simulink model "driver"  (R2013a)
settings: Solver=ode3  SolverMode=SingleTasking  StartTime=0.0  StopTime=inf  RelTol=1e-3
StartFcn:
  | %The GUI handles are by default hidden, turn them on
  | set(0,'ShowHiddenHandles','on');
  | 
  | %event listener for color detector
  | blk = 'driver/Color Detector/detector';
  | event = 'PostOutputs';
  | listener = @update_gui_circle_detect;
  | h = add_exec_event_listener(blk, event, listener);
  | 
  | %event listener for steering angle (manual drive)
  | blk2 = 'driver/Encoder1';
  | event2 = 'PostOutputs';
  | listener2 = @update_gui_steer_angle;
  | h2 = add_exec_event_listener(blk2, event2, listener2);
  | 
  | %event listener for pose updates
  | blk3 = 'driver/Dead Reckoning/Bicycle Model/Pose Integrator';
  | event3 = 'PostOutputs';
  | listener3 = @update_gui_robot_pose;
  | h3 = add_exec_event_listener(blk3, event3, listener3);
undefined symbols (not defined in the file or in its folder): Normalized, PARAMS
libraries: legonxtlib x8, simulink x1
settings Model: SimulationMode=external  ExtModeTrigDuration=2  Creator=anton  LastModifiedBy=anton
settings OptimizationCC: OptimizeModelRefInitCode=on  LifeSpan=1
settings DebuggingCC: SolverPrmCheckMsg=none  StrictBusMsg=Warning
settings HardwareCC: ProdLargestAtomicInteger=Long  ProdLargestAtomicFloat=Float  ProdEndianess=LittleEndian  ProdHWDeviceType=ARM Compatible->ARM 7
settings RTWCC: SystemTargetFile=realtime.tlc  GenerateMakefile=off  TemplateMakefile=realtime.tmf  Description=Run on Target Hardware  RTWVerbose=off  ProcessScript=realtime_make_rtw_hook
settings STFCustomTargetCC: TargetLibSuffix=.a  GenerateSampleERTMain=on  ERTCustomFileBanners=on  SupportNonInlinedSFcns=off  SupportVariableSizeSignals=on  MATLABClassNameForMDSCustomization=Simulink.SoftwareTarget.ERTCustomization  SystemTargetFile=realtime.tlc
settings ERTTargetCC: ParMdlRefBuildCompliant=off  CompOptLevelCompliant=off  ConcurrentExecutionCompliant=off  CombineOutputUpdateFcns=off  ERTFirstTimeCompliant=off  SupportContinuousTime=on  SupportVariableSizeSignals=on  ModelStepFunctionPrototypeControlCompliant=off  CPPClassGenCompliant=off  ExtMode=on  ExtModeTransport=2  ExtModeMexFile=ext_serial_win32_comm_no_acks_rtt  ExtModeMexArgs=0 5 9600  ERTSrcFileBannerTemplate=realtime_code_template.cgt  ERTHdrFileBannerTemplate=realtime_code_template.cgt  ERTDataSrcFileTemplate=realtime_code_template.cgt  ERTDataHdrFileTemplate=realtime_code_template.cgt  ERTCustomFileTemplate=realtime_file_process.tlc

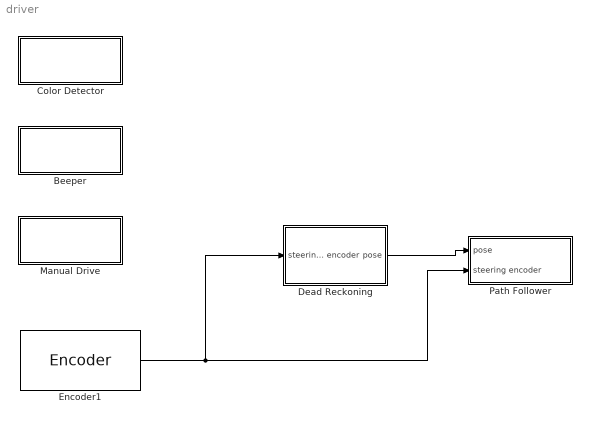
== system driver ==
  Beeper : Subsystem
  Color Detector : Subsystem
  Dead Reckoning : Subsystem
  Encoder1 : legonxtlib/Encoder  portNumber=A  opMode=No reset  sampleTime=0.01
  Manual Drive : Subsystem
  Path Follower : Subsystem
  wires:
  Dead Reckoning/1(pose) -> Path Follower/1(pose)
  Encoder1/1 -> Path Follower/2(steering encoder), Dead Reckoning/1(steering encoder)

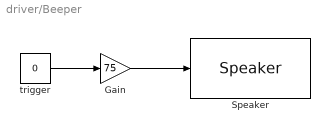
== system driver/Beeper ==
  Gain : Gain  Gain=75
  Speaker : legonxtlib/Speaker  sinputMode=Volume only  sspeakerFreq=440  sspeakerVolume=50  sspeakerDuration=50
  trigger : Constant  Value=0
  wires:
  Gain/1 -> Speaker/1
  trigger/1 -> Gain/1

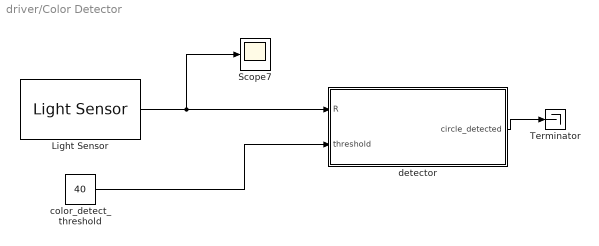
== system driver/Color Detector ==
  Light Sensor : legonxtlib/Light Sensor  portNumber=1  outputMode=Normalized (0 -100)  lightOn=on  sampleTime=0.1
  Scope7 : Scope
      settings: YMin=25  YMax=65
  Terminator : Terminator
  color_detect_threshold : Constant  Value=40
  detector : MATLAB Function  TreatAsAtomicUnit=on
  wires:
  detector/1(circle_detected) -> Terminator/1
  color_detect_threshold/1 -> detector/2(threshold)
  Light Sensor/1 -> Scope7/1, detector/1(R)

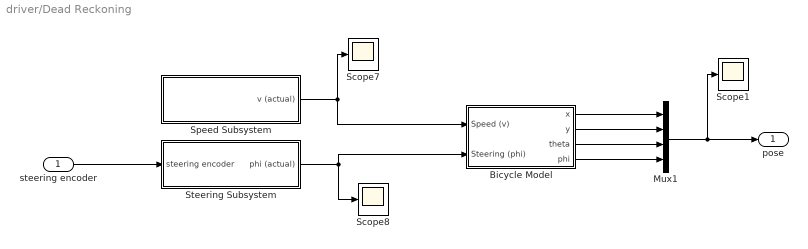
== system driver/Dead Reckoning ==
  steering encoder : Inport
  Bicycle Model : Subsystem
  Mux1 : Mux
  Scope1 : Scope
      settings: YMin=0  YMax=0.95
  Scope7 : Scope
      settings: YMin=0  YMax=14  SaveName=ScopeData19
  Scope8 : Scope
      settings: YMin=0.0523599  YMax=0.0523599  SaveName=ScopeData20
  Speed Subsystem : Subsystem
  Steering Subsystem : Subsystem
  pose : Outport
  wires:
  Bicycle Model/2(y) -> Mux1/2
  Bicycle Model/1(x) -> Mux1/1
  Bicycle Model/3(theta) -> Mux1/3
  Steering Subsystem/1(phi (actual)) -> Scope8/1, Bicycle Model/2(Steering (phi))
  Speed Subsystem/1(v (actual)) -> Bicycle Model/1(Speed (v)), Scope7/1
  Bicycle Model/4(phi) -> Mux1/4
  Mux1/1 -> Scope1/1, pose/1
  steering encoder/1 -> Steering Subsystem/1(steering encoder)

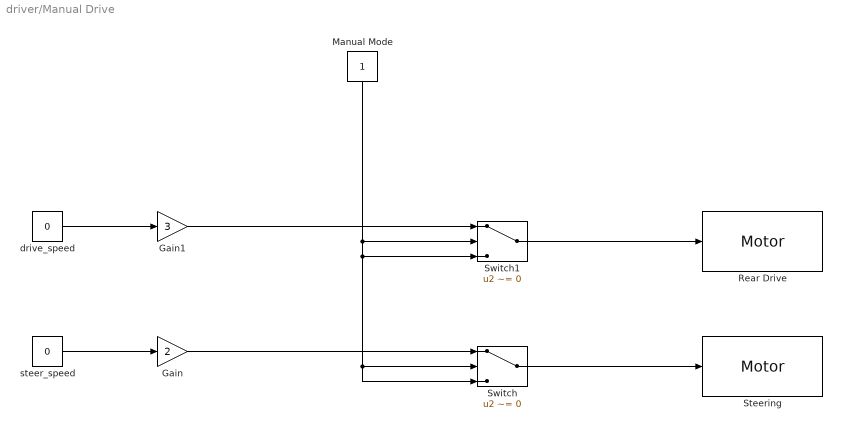
== system driver/Manual Drive ==
  Gain : Gain  Gain=2
  Gain1 : Gain  Gain=3
  Manual Mode : Constant
  Rear Drive : legonxtlib/Motor  sportNumber=C  sstopAction=Brake
  Steering : legonxtlib/Motor  sportNumber=A  sstopAction=Brake
  Switch : Switch  Criteria=u2 ~= 0
  Switch1 : Switch  Criteria=u2 ~= 0
  drive_speed : Constant  Value=0
  steer_speed : Constant  Value=0
  wires:
  Switch/1 -> Steering/1
  Switch1/1 -> Rear Drive/1
  steer_speed/1 -> Gain/1
  drive_speed/1 -> Gain1/1
  Gain/1 -> Switch/1
  Gain1/1 -> Switch1/1
  Manual Mode/1 -> Switch/3, Switch/2, Switch1/3, Switch1/2

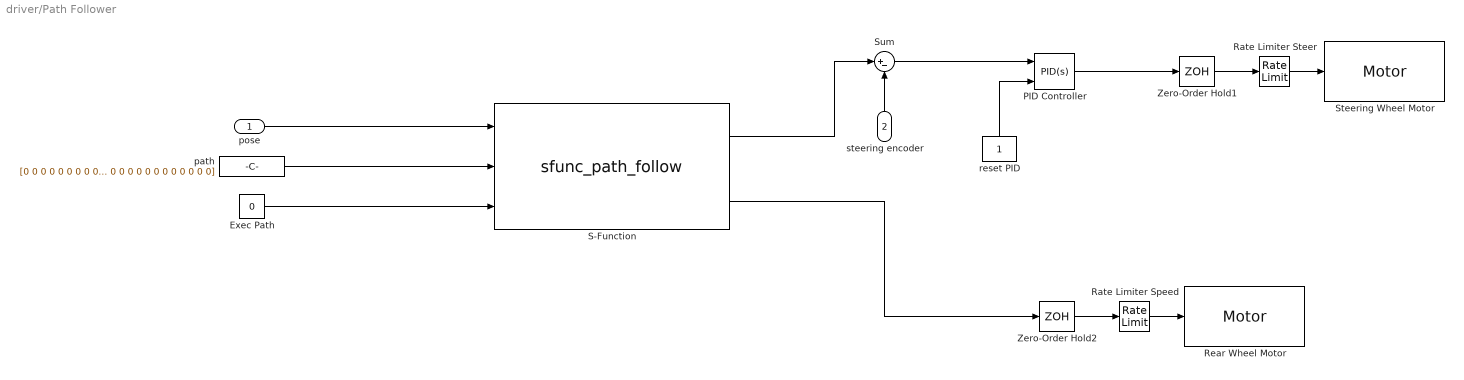
== system driver/Path Follower ==
  pose : Inport
  steering encoder : Inport  Port=2
  Exec Path : Constant  Value=0
  PID Controller : simulink/Continuous/PID Controller  Controller=PID  TimeDomain=Continuous-time  SampleTime=1  IntegratorMethod=Forward Euler  FilterMethod=Forward Euler  Form=Parallel  P=1  I=1  D=0  N=100  InitialConditionSource=internal  InitialConditionForIntegrator=0  InitialConditionForFilter=0  ExternalReset=either  LimitOutput=off  UpperSaturationLimit=inf  LowerSaturationLimit=-inf  LinearizeAsGain=on  AntiWindupMode=none  Kb=1  TrackingMode=off  Kt=1  PParamMin=[]  PParamMax=[]  IParamMin=[]  IParamMax=[]  DParamMin=[]  DParamMax=[]  NParamMin=[]  NParamMax=[]  KbParamMin=[]  KbParamMax=[]  KtParamMin=[]  KtParamMax=[]  POutMin=[]  POutMax=[]  IOutMin=[]  IOutMax=[]  DOutMin=[]  DOutMax=[]  NOutMin=[]  NOutMax=[]  KbOutMin=[]  KbOutMax=[]  KtOutMin=[]  KtOutMax=[]  IntegratorOutMin=[]  IntegratorOutMax=[]  FilterOutMin=[]  FilterOutMax=[]  SumOutMin=[]  SumOutMax=[]  SumI1OutMin=[]  SumI1OutMax=[]  SumI2OutMin=[]  SumI2OutMax=[]  SumI3OutMin=[]  SumI3OutMax=[]  SumDOutMin=[]  SumDOutMax=[]  SaturationOutMin=[]  SaturationOutMax=[]  IntegratorContinuousStateAttributes=''  IntegratorStateMustResolveToSignalObject=off  IntegratorRTWStateStorageClass=Auto  FilterContinuousStateAttributes=''  FilterStateMustResolveToSignalObject=off  FilterRTWStateStorageClass=Auto
  Rate Limiter Speed : RateLimiter  RisingSlewLimit=5  FallingSlewLimit=-5  SampleTimeMode=inherited
  Rate Limiter Steer : RateLimiter  RisingSlewLimit=5  FallingSlewLimit=-5  SampleTimeMode=inherited
  Rear Wheel Motor : legonxtlib/Motor  sportNumber=C  sstopAction=Brake
  S-Function : S-Function  FunctionName=sfunc_path_follow  SFunctionModules=sfunc_path_follow_wrapper  EnableBusSupport=off
      mask init:
      | val = [[.9  0.75 0.75 1 1 .9 .9 1]',[1 1 0.75 0.75 .9 .9 1 .9]'];try , sys = get_param(gcb,'SfunBuilderFcnName');if isempty(sys), sys = get_param(gcb,'FunctionName'); end,catch, sys = get_param(gcb,'FunctionName'); end
      settings: PreSaveFcn=try, set_param(gcb,'FunctionName','sfunc_path_follow'), end
      mask Display: plot(val(:,1),val(:,2)),disp(sys), port_label('input',1,'pose'), port_label('input',2,'path'), port_label('input',3,'exec_path'), port_label('output',1,'steer_angle'), port_label('output',2,'drive_speed')
  Steering Wheel Motor : legonxtlib/Motor  sportNumber=A  sstopAction=Brake
  Sum : Sum  Inputs=|+-
  Zero-Order Hold1 : ZeroOrderHold  SampleTime=0.01
  Zero-Order Hold2 : ZeroOrderHold  SampleTime=0.01
  path : Constant  Value=[0 0 0 0 0 0 0 0 0 0 0 0 0 0 0 0 0 0 0 0;0 0 0 0 0 0 0 0 0 0 0 0 0 0 0 0 0 0 0 0;0 0 0 0 0 0 0 0 0 0 0 0 0 0 0 0 0 0 0 0;0 0 0 0 0 0 0 0 0 0 0 0 0 0 0 0 0 0 0 0;0 0 0 0 0 0 0 0 0 0 0 0 0 0 0 0 0 0 0 0;0 0 0 0 0 0 0 0 0 0 0 0 0 0 0 0 0 0 0 0]  VectorParams1D=off
  reset PID : Constant
  wires:
  Zero-Order Hold1/1 -> Rate Limiter Steer/1
  Rate Limiter Steer/1 -> Steering Wheel Motor/1
  Rate Limiter Speed/1 -> Rear Wheel Motor/1
  Zero-Order Hold2/1 -> Rate Limiter Speed/1
  pose/1 -> S-Function/1
  S-Function/2 -> Zero-Order Hold2/1
  path/1 -> S-Function/2
  Exec Path/1 -> S-Function/3
  S-Function/1 -> Sum/1
  Sum/1 -> PID Controller/1
  steering encoder/1 -> Sum/2
  reset PID/1 -> PID Controller/2
  PID Controller/1 -> Zero-Order Hold1/1

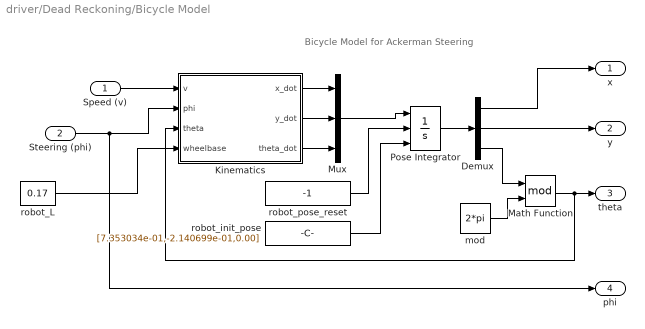
== system driver/Dead Reckoning/Bicycle Model ==
  note: Bicycle Model for Ackerman Steering
  Speed (v) : Inport
  Steering (phi) : Inport  Port=2
  Demux : Demux  Outputs=3
  Kinematics : MATLAB Function  TreatAsAtomicUnit=on
  Math Function : Math  Operator=mod  SaturateOnIntegerOverflow=on
  Mux : Mux  Inputs=3
  Pose Integrator : Integrator  ExternalReset=either  InitialConditionSource=external  InitialCondition=PARAMS.ROBOT_INIT_POSE
  mod : Constant  Value=2*pi
  robot_L : Constant  Value=0.17
  robot_init_pose : Constant  Value=[7.353034e-01,-2.140699e-01,0.00]
  robot_pose_reset : Constant  Value=-1
  x : Outport
  y : Outport  Port=2
  theta : Outport  Port=3
  phi : Outport  Port=4
  wires:
  Speed (v)/1 -> Kinematics/1(v)
  Steering (phi)/1 -> phi/1, Kinematics/2(phi)
  mod/1 -> Math Function/2
  Math Function/1 -> Kinematics/3(theta), theta/1
  Kinematics/1(x_dot) -> Mux/1
  Kinematics/2(y_dot) -> Mux/2
  Kinematics/3(theta_dot) -> Mux/3
  Mux/1 -> Pose Integrator/1
  robot_pose_reset/1 -> Pose Integrator/2
  Pose Integrator/1 -> Demux/1
  Demux/1 -> x/1
  Demux/2 -> y/1
  Demux/3 -> Math Function/1
  robot_L/1 -> Kinematics/4(wheelbase)
  robot_init_pose/1 -> Pose Integrator/3

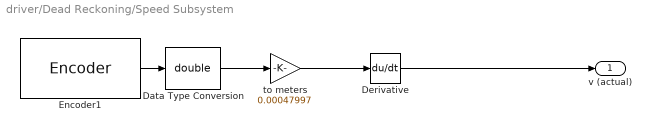
== system driver/Dead Reckoning/Speed Subsystem ==
  Data Type Conversion : DataTypeConversion  OutDataTypeStr=double  SaturateOnIntegerOverflow=on  RndMeth=Zero
  Derivative : Derivative
  Encoder1 : legonxtlib/Encoder  portNumber=C  opMode=No reset  sampleTime=0.01
  to meters : Gain  Gain=0.00047997
  v (actual) : Outport
  wires:
  Encoder1/1 -> Data Type Conversion/1
  Data Type Conversion/1 -> to meters/1
  to meters/1 -> Derivative/1
  Derivative/1 -> v (actual)/1

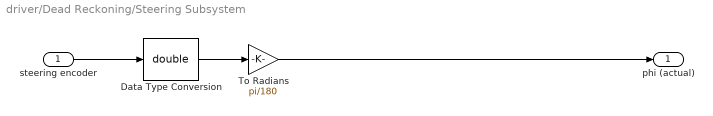
== system driver/Dead Reckoning/Steering Subsystem ==
  steering encoder : Inport
  Data Type Conversion : DataTypeConversion  OutDataTypeStr=double  SaturateOnIntegerOverflow=on  RndMeth=Zero
  To Radians : Gain  Gain=pi/180
  phi (actual) : Outport
  wires:
  Data Type Conversion/1 -> To Radians/1
  steering encoder/1 -> Data Type Conversion/1
  To Radians/1 -> phi (actual)/1

== matlab function driver/Dead Reckoning/Bicycle Model/Kinematics ==
  data: v input; x_dot output; y_dot output; theta_dot output; phi input; theta input; wheelbase input
function [x_dot, y_dot, theta_dot] = fcn(v, phi, theta, wheelbase)
    
    
    x_dot = v * cos(theta);
    y_dot = v * sin(theta);
    theta_dot = (v/wheelbase) * tan(phi);

== matlab function driver/Color Detector/detector ==
  data: R input; circle_detected output; threshold input
function circle_detected = fcn(R, threshold)

% we want to detect whether the robot is over a black patch. for this, just
% check whether all the R,G, and B values are under a given threshold.
% intensities are between 0-255.

    if (R < threshold)
        circle_detected = true;
    else
        circle_detected = false;
    end
